simulink model "sim2_nonmininum"  (R2018a)
settings: Solver=VariableStepAuto  StartTime=0.0  StopTime=60  RelTol=1e-3
values from neighbouring files (symbols this model uses):
  A = [-dG(2:end)',[1;0]]    [ex1_liu.m]    (also in ex2_fu.m; ex2_liu.m; ex3_geng.m; ex3_liu_geso.m)
  B = nG(2:end)'    [ex1_liu.m]    (also in ex2_fu.m; ex2_liu.m; ex3_geng.m; ex3_liu_geso.m)
  K = [0 1]*inv(Mx)*PcA    [ex1_liu.m]    (also in ex2_fu.m = acker(A,B,[p1 p2]); ex2_liu.m; ex3_geng.m = acker(A,B,[p1 p2]); ex3_liu_geso.m = place(A,B,[p1 p2]))
  kr = inv(C*inv(eye(2)-A+B*K)*B)    [ex1_liu.m]    (also in ex2_fu.m = inv([1 0]*inv(eye(2)-A+B*K)*B); ex2_liu.m; ex3_geng.m = inv([1 0]*inv(eye(2)-A+B*K)*B); ex3_liu_geso.m = inv([1 0]*inv(eye(2)-A+B*K)*B))
  Ts = 0.1    [ex1_liu.m]    (also in ex2_fu.m = 0.05; ex2_liu.m; ex3_geng.m = 0.01; gerar_figuras.m)
libraries: cstblocks x8, simulink x2
settings Model: Creator=Bismark  LastModifiedBy=Dell

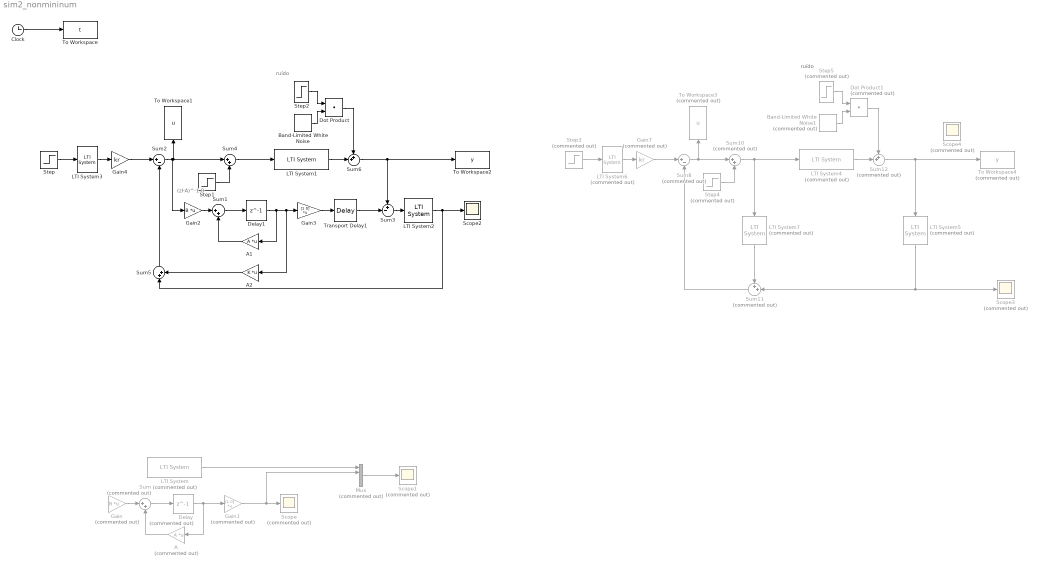
== system sim2_nonmininum ==
  note: ruído
  note: (zI-A)^-1.B
  note: ruído
  A : Gain  Commented=on  Gain=A  Multiplication=Matrix(K*u) (u vector)
  A1 : Gain  Gain=A  Multiplication=Matrix(K*u) (u vector)
  A2 : Gain  Gain=K  Multiplication=Matrix(K*u) (u vector)
  Band-Limited White Noise : simulink/Sources/Band-Limited White Noise  Cov=[0.00001]  Ts=Ts  seed=[23341]
  Band-Limited White Noise1 : simulink/Sources/Band-Limited White Noise  Commented=on  Cov=[0.00001]  Ts=Ts  seed=[23341]
  Clock : Clock
  Delay : Delay  Commented=on  DelayLength=1  SampleTime=Ts
  Delay1 : Delay  DelayLength=1  SampleTime=Ts
  Dot Product : DotProduct  InputSameDT=on  OutDataTypeStr=Inherit: Inherit via internal rule
  Dot Product1 : DotProduct  Commented=on  InputSameDT=on  OutDataTypeStr=Inherit: Inherit via internal rule
  Gain : Gain  Commented=on  Gain=B  Multiplication=Matrix(K*u) (u vector)
  Gain1 : Gain  Commented=on  Gain=[1 0]  Multiplication=Matrix(K*u)
  Gain2 : Gain  Gain=B  Multiplication=Matrix(K*u) (u vector)
  Gain3 : Gain  Gain=[1 0]  Multiplication=Matrix(K*u)
  Gain4 : Gain  Gain=kr
  Gain7 : Gain  Commented=on  Gain=kr
  LTI System : cstblocks/LTI System  Commented=on  sys=G  IC=[]
  LTI System1 : cstblocks/LTI System  sys=Pr  IC=[]
  LTI System2 : cstblocks/LTI System  sys=V  IC=[]
  LTI System3 : cstblocks/LTI System  sys=Fr  IC=[]
  LTI System4 : cstblocks/LTI System  Commented=on  sys=Pr  IC=[]
  LTI System5 : cstblocks/LTI System  Commented=on  sys=V  IC=[]
  LTI System6 : cstblocks/LTI System  Commented=on  sys=Fr  IC=[]
  LTI System7 : cstblocks/LTI System  Commented=on  sys=S  IC=[]
  Mux : Mux  Commented=on
  Scope{,1,3..4} (4 alike) : Scope  Commented=on
  Scope2 : Scope
  Step : Step  Time=0  SampleTime=0
  Step1 : Step  Time=30  After=-1  SampleTime=Ts
  Step2 : Step  Time=55  SampleTime=0
  Step3 : Step  Commented=on  Time=0  SampleTime=0
  Step4 : Step  Commented=on  Time=30  After=-1  SampleTime=Ts
  Step5 : Step  Commented=on  Time=55  SampleTime=0
  Sum : Sum  Commented=on  Inputs=|++
  Sum1 : Sum  Inputs=|++
  Sum10 : Sum  Commented=on  Inputs=|++
  Sum11 : Sum  Commented=on  Inputs=++|
  Sum12 : Sum  Commented=on  Inputs=++|
  Sum2 : Sum  Inputs=|+-
  Sum3 : Sum  Inputs=+-|
  Sum4 : Sum  Inputs=|++
  Sum5 : Sum  Inputs=|++
  Sum6 : Sum  Inputs=++|
  Sum8 : Sum  Commented=on  Inputs=|+-
  To Workspace : ToWorkspace  VariableName=t  SampleTime=Ts
  To Workspace1 : ToWorkspace  VariableName=u  SampleTime=Ts
  To Workspace2 : ToWorkspace  VariableName=y  SampleTime=Ts
  To Workspace3 : ToWorkspace  Commented=on  VariableName=u  SampleTime=Ts
  To Workspace4 : ToWorkspace  Commented=on  VariableName=y  SampleTime=Ts
  Transport Delay1 : TransportDelay
  wires:
  Step/1 -> LTI System3/1
  Delay1/1 -> A1/1, A2/1, Gain3/1
  Sum1/1 -> Delay1/1
  Gain2/1 -> Sum1/1
  A1/1 -> Sum1/2
  Sum2/1 -> Gain2/1, Sum4/1, To Workspace1/1
  Gain4/1 -> Sum2/1
  Clock/1 -> To Workspace/1
  Gain3/1 -> Transport Delay1/1
  Transport Delay1/1 -> Sum3/2
  Sum4/1 -> LTI System1/1
  Step1/1 -> Sum4/2
  Sum6/1 -> Sum3/1, To Workspace2/1
  Sum5/1 -> Sum2/2
  A2/1 -> Sum5/2
  Sum3/1 -> LTI System2/1
  LTI System2/1 -> Scope2/1, Sum5/1
  LTI System3/1 -> Gain4/1
  Step2/1 -> Dot Product/1
  Band-Limited White Noise/1 -> Dot Product/2
  Dot Product/1 -> Sum6/1
  LTI System1/1 -> Sum6/2
  Gain1/1 -> Mux/2, Scope/1
  Mux/1 -> Scope1/1
  A/1 -> Sum/2
  Sum/1 -> Delay/1
  Delay/1 -> A/1, Gain1/1
  Gain/1 -> Sum/1
  LTI System/1 -> Mux/1
  LTI System5/1 -> Sum11/2, Scope3/1
  Gain7/1 -> Sum8/1
  Step4/1 -> Sum10/2
  Sum12/1 -> LTI System5/1, To Workspace4/1
  Dot Product1/1 -> Sum12/1
  LTI System4/1 -> Sum12/2
  Band-Limited White Noise1/1 -> Dot Product1/2
  Step3/1 -> LTI System6/1
  Step5/1 -> Dot Product1/1
  LTI System6/1 -> Gain7/1
  Sum8/1 -> Sum10/1, To Workspace3/1
  Sum11/1 -> Sum8/2
  LTI System7/1 -> Sum11/1
  Sum10/1 -> LTI System7/1, LTI System4/1
